simulink model "encoder_hall_block1"  (R2012b)
settings: Solver=ode45  StartTime=0.0  StopTime=3*pi  FixedStep=1e-5  MaxStep=1e-3  RelTol=1e-3
libraries: Encoder x1
settings Model: Creator=h3now  LastModifiedBy=h3now

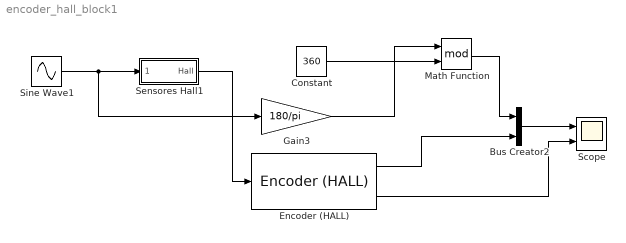
== system encoder_hall_block1 ==
  Bus Creator2 : BusCreator  Inputs=2
  Constant : Constant  Value=360
  Encoder (HALL) : Encoder/Encoder (HALL)
  Gain3 : Gain  Gain=180/pi
  Math Function : Math  Operator=mod  SaturateOnIntegerOverflow=on
  Scope : Scope  NumInputPorts=2
      settings: YMin=-5~-5  YMax=5~5  SaveName=ScopeData7
  Sensores Hall1 : Subsystem
  Sine Wave1 : Sin  Amplitude=2*pi  SampleTime=0
  wires:
  Sine Wave1/1 -> Sensores Hall1/1(teta_e), Gain3/1
  Sensores Hall1/1(Hall) -> Encoder (HALL)/1
  Encoder (HALL)/1 -> Bus Creator2/2
  Bus Creator2/1 -> Scope/1
  Gain3/1 -> Math Function/1
  Constant/1 -> Math Function/2
  Math Function/1 -> Bus Creator2/1
  Encoder (HALL)/2 -> Scope/2

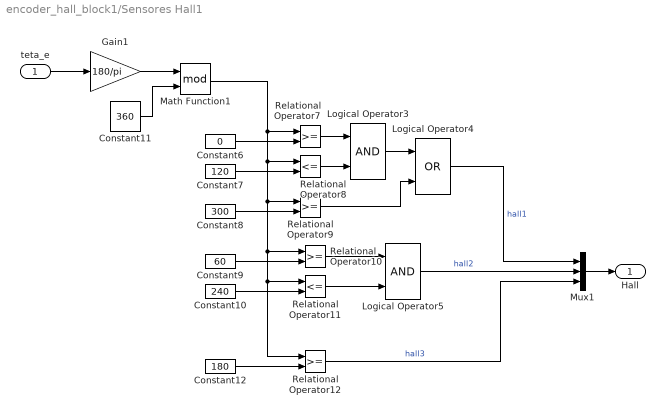
== system encoder_hall_block1/Sensores Hall1 ==
  teta_e : Inport
  Constant10 : Constant  Value=240
  Constant11 : Constant  Value=360
  Constant12 : Constant  Value=180
  Constant6 : Constant  Value=0
  Constant7 : Constant  Value=120
  Constant8 : Constant  Value=300
  Constant9 : Constant  Value=60
  Gain1 : Gain  Gain=180/pi
  Logical Operator3 : Logic  AllPortsSameDT=off  OutDataTypeStr=boolean
  Logical Operator4 : Logic  Operator=OR  AllPortsSameDT=off  OutDataTypeStr=boolean
  Logical Operator5 : Logic  AllPortsSameDT=off  OutDataTypeStr=boolean
  Math Function1 : Math  Operator=mod  SaturateOnIntegerOverflow=on
  Mux1 : Mux  Inputs=3
  Relational Operator{7,9..10,12} (4 alike) : RelationalOperator  InputSameDT=on
  Relational Operator11 : RelationalOperator  Operator=<=  InputSameDT=on
  Relational Operator8 : RelationalOperator  Operator=<=  InputSameDT=on
  Hall : Outport
  wires:
  Math Function1/1 -> Relational Operator7/1, Relational Operator12/1, Relational Operator11/1, Relational Operator10/1, Relational Operator9/1, Relational Operator8/1
  Constant11/1 -> Math Function1/2
  Gain1/1 -> Math Function1/1
  Relational Operator12/1 -> Mux1/3  "hall3"
  Logical Operator5/1 -> Mux1/2  "hall2"
  Logical Operator4/1 -> Mux1/1  "hall1"
  Mux1/1 -> Hall/1
  Constant12/1 -> Relational Operator12/2
  Constant10/1 -> Relational Operator11/2
  Constant9/1 -> Relational Operator10/2
  Relational Operator11/1 -> Logical Operator5/2
  Relational Operator10/1 -> Logical Operator5/1
  Relational Operator8/1 -> Logical Operator3/2
  Relational Operator7/1 -> Logical Operator3/1
  Logical Operator3/1 -> Logical Operator4/1
  Relational Operator9/1 -> Logical Operator4/2
  Constant8/1 -> Relational Operator9/2
  Constant7/1 -> Relational Operator8/2
  Constant6/1 -> Relational Operator7/2
  teta_e/1 -> Gain1/1
